simulink model "Vorlage_Bilder"  (R2016a)
settings: Solver=VariableStepAuto  StartTime=0.0  StopTime=10.0  RelTol=1e-3
undefined symbols (not defined in the file): K_yz, T_x_AP, x_0_yz, x_AP
libraries: simulink x1
settings Model: Creator=Florian  LastModifiedBy=Florian

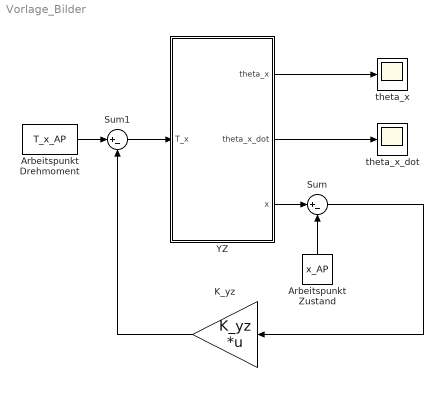
== system Vorlage_Bilder ==
  Arbeitspunkt Zustand : Constant  Value=x_AP
  Arbeitspunkt Drehmoment : Constant  Value=T_x_AP
  K_yz : Gain  Gain=K_yz  Multiplication=Matrix(K*u) (u vector)
  Sum : Sum  Inputs=|+-
  Sum1 : Sum  Inputs=|+-
  YZ : Subsystem
  theta_x : Scope
  theta_x_dot : Scope
  wires:
  Arbeitspunkt Drehmoment/1 -> Sum1/1
  Arbeitspunkt Zustand/1 -> Sum/2
  YZ/3(x) -> Sum/1
  Sum1/1 -> YZ/1("T_x ")
  K_yz/1 -> Sum1/2
  Sum/1 -> K_yz/1
  YZ/1(theta_x) -> theta_x/1
  YZ/2(theta_x_dot) -> theta_x_dot/1

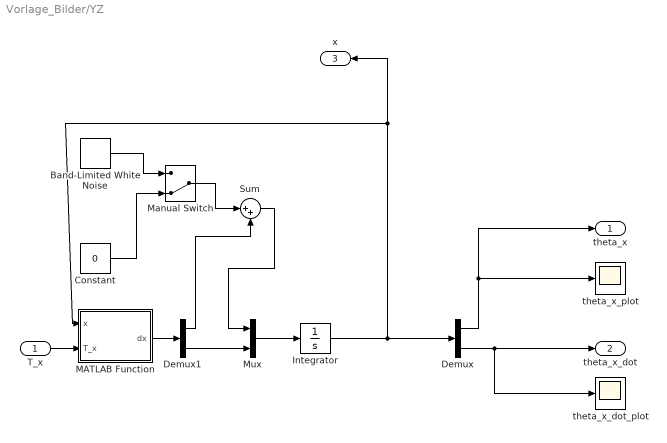
== system Vorlage_Bilder/YZ ==
  "T_x " : Inport
  Band-Limited White Noise : simulink/Sources/Band-Limited White Noise  Cov=[0.1^2]  Ts=1/92  seed=[23341]
  Constant : Constant  Value=0
  Demux : Demux  Outputs=2
  Demux1 : Demux  Outputs=2
  Integrator : Integrator  InitialCondition=x_0_yz
  MATLAB Function : MATLAB Function  TreatAsAtomicUnit=on
  Manual Switch : ManualSwitch  CurrentSetting=0
  Mux : Mux  Inputs=2
  Sum : Sum  Inputs=|++
  theta_x_dot_plot : Scope
  theta_x_plot : Scope
  theta_x : Outport
  theta_x_dot : Outport  Port=2
  x : Outport  Port=3
  wires:
  Demux/1 -> theta_x/1, theta_x_plot/1
  MATLAB Function/1(dx) -> Demux1/1
  Mux/1 -> Integrator/1
  "T_x "/1 -> MATLAB Function/2(T_x)
  Demux/2 -> theta_x_dot/1, theta_x_dot_plot/1
  Manual Switch/1 -> Sum/1
  Band-Limited White Noise/1 -> Manual Switch/1
  Constant/1 -> Manual Switch/2
  Integrator/1 -> MATLAB Function/1(x), x/1, Demux/1
  Demux1/2 -> Mux/2
  Demux1/1 -> Sum/2
  Sum/1 -> Mux/1

== matlab function Vorlage_Bilder/YZ/MATLAB Function ==
  data: x input; T_x input; dx output

function dx = fcn(x,T_x)

%Zuweisung Koordinaten und Ableitungen
theta_x=x(1);
theta_x_dot=x(2);



theta_x_dotdot = -(21954653710653549407969203978240000000*T_x - 210647080406124048865923105508646977536*sin(theta_x) - 1439521453041267026494975497910312500*theta_x_dot^2*sin(theta_x) + 109694540352150173612405046640640000000*T_x*cos(theta_x) + 1390470442377399145148585068800234375*theta_x_dot^2*cos(theta_x)*sin(theta_x))/(234375*(12283916399285478626090457582168*cos(theta_x) - 5932673887476903019300629626881*cos(theta_x)^2 + 46171199208284847673663943663264));




%Zuweisung Ausgang
dx = [theta_x_dot; theta_x_dotdot];
end
